simulink model "harmonic_motion"  (R2019b)
settings: Solver=VariableStepAuto  StartTime=0.0  StopTime=30  RelTol=1e-3
settings Model: Creator=Shiwei Pan  LastModifiedBy=Shiwei Pan

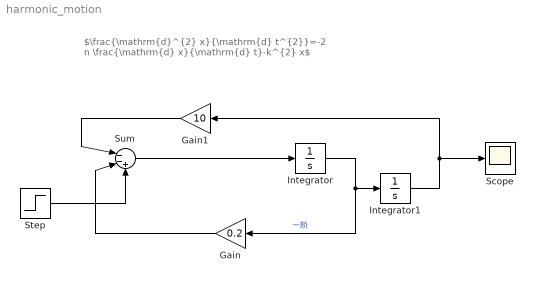
== system harmonic_motion ==
  note: $\frac{\mathrm{d}^{2} x}{\mathrm{d} t^{2}}=-2 n \frac{\mathrm{d} x}{\mathrm{d} t}-k^{2} x$
  Gain : Gain  Gain=0.2
  Gain1 : Gain  Gain=10
  Integrator : Integrator
  Integrator1 : Integrator
  Scope : Scope
  Step : Step  Time=0  After=20  SampleTime=0.01
  Sum : Sum  Inputs=|--+
  wires:
  Integrator/1 -> Gain/1, Integrator1/1  "一阶"
  Integrator1/1 -> Gain1/1, Scope/1
  Gain1/1 -> Sum/1
  Sum/1 -> Integrator/1
  Step/1 -> Sum/3
  Gain/1 -> Sum/2
